simulink model "MicrochipTargetMotorControl"  (R2024b)
settings: Solver=FixedStepDiscrete  StartTime=0.0  StopTime=50  RelTol=1e-3  EnableMultiTasking=on
InitFcn:
  | MicrochipTargetMotorControlData;
  | mcbMotorSwapData;
values from neighbouring files (symbols this model uses):
  Ts = T_pwm    [mcbMotorSwapData.m]
  Ts_motor = T_pwm/2    [mcbMotorSwapData.m]
  Ts_serialIn = 50e-3    (= 0.05)    [MicrochipTargetMotorControlData.m]
  Ts_speed = 10*Ts    [mcbMotorSwapData.m]
undefined symbols (not defined in the file or in its folder): A4, B0, C10, C11, C6, C7, C8, inverter, MaxPer, P17, P20, P39, P40, P41, P43, P44, Pin, pmsm, Resol, s, target, Timer, us
libraries: MCHP_Blockset x19, simulink x13, autolibpmsminterior x1, mcbplantlib x1, mcbcontrolslib x1
(part 1 of 4)
settings Model: ExtModeEnableFloating=off  ExtModeTrigDuration=20  Creator=Lubin Kerhuel  LastModifiedBy=snarayan
settings SolverCC: AlgebraicLoopSolver=TrustRegion
settings OptimizationCC: DefaultParameterBehavior=Inlined  DefaultUnderspecifiedDataType=single  InlineInvariantSignals=on  StrengthReduction=on  PassReuseOutputArgsAs=Individual arguments  ZeroExternalMemoryAtStartup=off  ZeroInternalMemoryAtStartup=off  OptimizeBlockOrder=speed  OptimizationPriority=Speed  OptimizationCustomize=off  MultiThreadedLoops=on  AutoScheduleForLoops=on  EfficientTunableParamExpr=on
settings DebuggingCC: MultiTaskDSMMsg=none  MultiTaskCondExecSysMsg=none  MultiTaskRateTransMsg=warning  ParameterPrecisionLossMsg=none  ParameterTunabilityLossMsg=error  UnconnectedInputMsg=warning  UnconnectedOutputMsg=warning  UnconnectedLineMsg=warning  ArithmeticOperatorsInVariantConditions=warning
settings HardwareCC: ProdBitPerPointer=32  ProdBitPerSizeT=32  ProdBitPerPtrDiffT=32  ProdLargestAtomicInteger=Long  ProdWordSize=32  ProdHWDeviceType=Generic->Custom
settings ModelReferenceCC: ModelReferenceNumInstancesAllowed=Single
settings SFSimCC: MATLABDynamicMemAlloc=off  CustomCodeUndefinedFunction=UseInterfaceOnly
settings RTWCC: Description=Microchip Embedded Target dsPIC33A (real-time)  SystemTargetFile=MCHP_dsPIC33A_stf.tlc  TLCOptions="-aExtModeXCPClassicInterface=0  -aCreateExtModeTypes=1 -aExtModeXCPSimulationTimeInTicks=1"  TemplateMakefile=MCHP_dsPIC33A.tmf  GPUComputeCapability=3.5
settings RTWCC: CustomSourceCode=|
  | void DisablePWMOutputs(void)
  | {
  |     PG3IOCONbits.OVRDAT = 0;
  |     PG2IOCONbits.OVRDAT = 0;
  |     PG1IOCONbits.OVRDAT = 0;
  |     PG3IOCONbits.OVRENH = 1;
  |     PG3IOCONbits.OVRENL = 1;
  |     PG2IOCONbits.OVRENH = 1;
  |     PG2IOCONbits.OVRENL = 1;
  |     PG1IOCONbits.OVRENH = 1;
  |     PG1IOCONbits.OVRENL = 1;
  | }
  | 
  | 
  | void EnablePWMOutputs(void)
  | {
  |     PG3IOCONbits.OVRENH = 0;
  |     PG3IOCONbits.OVRENL = 0;
  |     PG2IOCONbits.OVRENH = 0;
  |     PG2IOCONbits.OVRENL = 0;
  |     PG1IOCONbits.OVRENH = 0;
  |     PG1IOCONbits.OVRENL = 0;
  | }
settings CodeAppCC: ForceParamTrailComments=on  IgnoreCustomStorageClasses=off  MaxIdLength=255  OperatorAnnotations=on  SimulinkDataObjDesc=on  SFDataObjDesc=on  InsertBlockDesc=on
settings STFCustomTargetCC: TargetLibSuffix=_lib.a  TargetLangStandard=C99 (ISO)  MultiwordLength=256  CombineOutputUpdateFcns=on  CombineSignalStateStructs=on  SuppressErrorStatus=on  ERTCustomFileBanners=on  SupportContinuousTime=off  RemoveResetFunc=on  MATLABClassNameForMDSCustomization=Simulink.SoftwareTarget.ERTCustomization  SystemTargetFile=MCHP_dsPIC33A_stf.tlc
settings ERTTargetCC: TargetLibSuffix=_lib.a  TargetLangStandard=C99 (ISO)  ParMdlRefBuildCompliant=off  CompOptLevelCompliant=off  ConcurrentExecutionCompliant=off  CombineSignalStateStructs=on  SuppressErrorStatus=on  SupportNonInlinedSFcns=on  ModelStepFunctionPrototypeControlCompliant=off  CPPClassGenCompliant=off  UseToolchainInfoCompliant=off  ExtModeTransport=1  ExtModeStaticAlloc=on  ExtModeStaticAllocSize=1024  ExtModeMexFile=ext_xcp  ExtModeMexArgs=1 0 460800 './mclv_48v_300w_dspic33ak128mc106_opticalencoder.X/mclv_48v_300w_dspic33ak128mc106_opticalencoder.elf'  ExtModeIntrfLevel=Level2 - Open  ERTSrcFileBannerTemplate=MCHP_dsPIC_code_template.cgt  ERTHdrFileBannerTemplate=MCHP_dsPIC_code_template.cgt  ERTDataSrcFileTemplate=MCHP_dsPIC_code_template.cgt  ERTDataHdrFileTemplate=MCHP_dsPIC_code_template.cgt  ERTCustomFileTemplate=MCHP_main.tlc  MaxLineWidth=110  DynamicArrayContainerType=coder::array

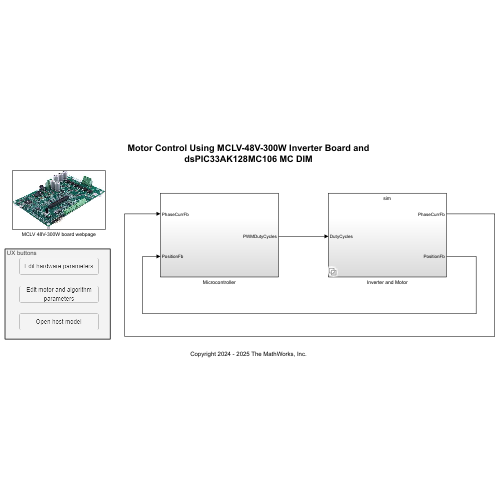
[thumbnail: Simulink's stored preview of the top-level diagram]
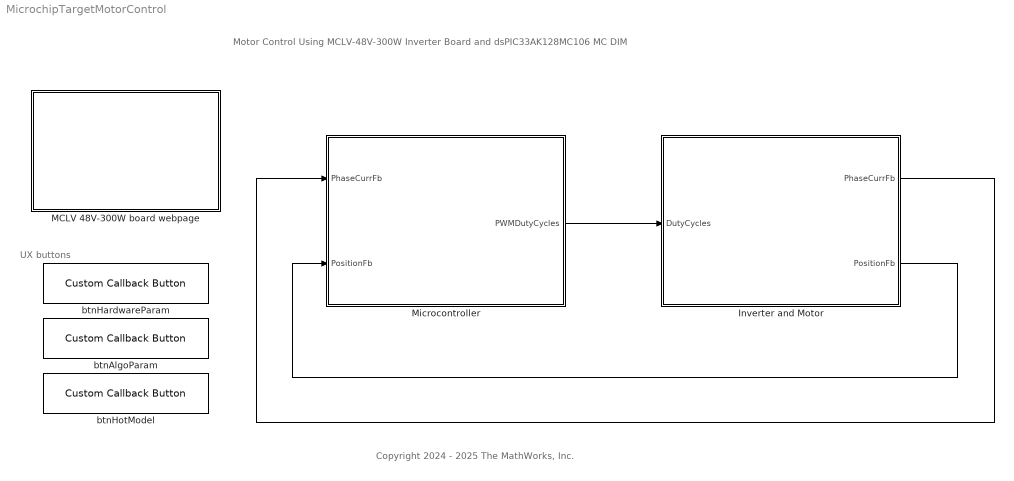
== system MicrochipTargetMotorControl ==
  note: Motor Control Using MCLV-48V-300W Inverter Board and dsPIC33AK128MC106 MC DIM
  note: UX buttons
  note: Copyright 2024 - 2025 The MathWorks, Inc.
  Inverter and Motor : Subsystem  Variant=on  VariantControlMode=sim codegen switching
  MCLV 48V-300W board webpage : Subsystem
      settings: OpenFcn=|
      | web('https://www.microchip.com/en-us/development-tool/EV62P66A','-browser'); % dsPIC33CK256MP508 DIM
      | pause(1);
      | web('https://www.microchip.com/en-us/development-tool/EV18H47A','-browser'); % LVMC 300W
      mask Display: image('MCHP_i_Board_MCLV_300W48V_reduced.jpg');
  Microcontroller : Subsystem
  btnAlgoParam : CustomCallbackButton  Configuration="{\"components\":[{\"name\":\"BackgroundImageComponent\",\"settings\":{\"image\":{\"size\":[0,0],\"src\":\"default\",\"srcOrientation\":\"Right\"},\"position\":[0,0,1,1]}},{\"name\":\"ButtonStateComponent\",\"settings\":{\"buttonType\":\"momentary\",\"clickFcn\":\"edit mcbMotorSwapData.m;\",\"onValue\":1,\"position\":[0,0,1,1],\"pressDelay\":\"500\",\"pressFcn\":\"\",\"repeatInterval\":\"0\",\"states\":[{\"horizontalAlignment\":\"center\",\"image\":{\"position\":[0,0,1,1],\"size\":[1,1],\"src\":\"default\",\"srcOrientation\":\"Right\"},\"label\":{\"color\":[0.01176470588,0.01176470588,0.01176470588,1],\"icon\":{\"size\":[0,0],\"src\":\"default\",\"srcOrientation\":\"Right\"},\"iconPlacement\":\"left\",\"opacity\":1,\"show\":true,\"text\":{\"content\":\"Edit motor and algorithm parameters\",\"font\":\"Helvetica\"}},\"labelOffset\":[0,0],\"verticalAlignment\":\"middle\"},{\"horizontalAlignment\":\"center\",\"image\":{\"position\":[0,0,1,1],\"size\":[1,1],\"src\":\"default\",\"srcOrientation\":\"Right\"},\"label\":{\"color\":[0.01176470588,0.01176470588,0.01176470588,1],\"icon\":{\"size\":[0,0],\"src\":\"default\",\"srcOrientation\":\"Right\"},\"iconPlacement\":\"left\",\"opacity\":1,\"show\":true,\"text\":{\"content\":\"Edit motor and algorithm parameters\",\"font\":\"Helvetica\"}},\"labelOffset\":[0,0],\"verticalAlignment\":\"middle\"},{\"horizontalAlignment\":\"center\",\"image\":{\"position\":[0,0,1,1],\"size\":[1,1],\"src\":\"default\",\"srcOrientation\":\"Right\"},\"label\":{\"color\":[0.01176470588,0.01176470588,0.01176470588,1],\"icon\":{\"size\":[0,0],\"src\":\"default\",\"srcOrientation\":\"Right\"},\"iconPlacement\":\"left\",\"opacity\":1,\"show\":true,\"text\":{\"content\":\"Edit motor and algorithm parameters\",\"font\":\"Helvetica\"}},\"labelOffset\":[0,0],\"verticalAlignment\":\"middle\"},{\"horizontalAlignment\":\"center\",\"image\":{\"position\":[0,0,1,1],\"size\":[1,1],\"src\":\"default\",\"srcOrientation\":\"Right\"},\"label\":{\"color\":[0.01176470588,0.01176470588,0.01176470588,1],\"icon\":{\"size\":[0,0],\"src\":\"default\",\"srcOrientation\":\"Right\"},\"iconPlacement\":\"left\",\"opacity\":1,\"show\":true,\"text\":{\"content\":\"Edit motor and algorithm parameters\",\"font\":\"Helvetica\"}},\"labelOffset\":[0,0],\"verticalAlignment\":\"middle\"}]}},{\"name\":\"ForegroundImageComponent\",\"settings\":{\"image\":{\"size\":[0,0],\"src\":\"default\",\"srcOrientation\":\"Right\"},\"isForeground\":1,\"position\":[0,0,1,1]}}],\"settings\":{\"BindingType\":\"standalone\",\"backgroundColor\":[244,244,244,1],\"backgroundOffset\":0.2,\"backgroundOpacity\":1,\"fixedAspectRatio\":\"off\",\"foregroundColor\":[0.01176470588,0.01176470588,0.01176470588,1],\"migratedFromLegacy\":true,\"useBackgroundColor\":true,\"variant\":\"callback\",\"version\":\"R2024b\"},\"type\":\"Button\"}"  CustomBackgroundColor="{\"color\":[0.9568627451,0.9568627451,0.9568627451],\"show\":true}"
  btnHardwareParam : CustomCallbackButton  Configuration="{\"components\":[{\"name\":\"BackgroundImageComponent\",\"settings\":{\"image\":{\"size\":[0,0],\"src\":\"default\",\"srcOrientation\":\"Right\"},\"position\":[0,0,1,1]}},{\"name\":\"ButtonStateComponent\",\"settings\":{\"buttonType\":\"momentary\",\"clickFcn\":\"edit MicrochipTargetMotorControlData.m;\",\"onValue\":1,\"position\":[0,0,1,1],\"pressDelay\":\"500\",\"pressFcn\":\"\",\"repeatInterval\":\"0\",\"states\":[{\"horizontalAlignment\":\"center\",\"image\":{\"position\":[0,0,1,1],\"size\":[1,1],\"src\":\"default\",\"srcOrientation\":\"Right\"},\"label\":{\"color\":[0.01176470588,0.01176470588,0.01176470588,1],\"icon\":{\"size\":[0,0],\"src\":\"default\",\"srcOrientation\":\"Right\"},\"iconPlacement\":\"left\",\"opacity\":1,\"show\":true,\"text\":{\"content\":\"Edit hardware parameters\",\"font\":\"Helvetica\"}},\"labelOffset\":[0,0],\"verticalAlignment\":\"middle\"},{\"horizontalAlignment\":\"center\",\"image\":{\"position\":[0,0,1,1],\"size\":[1,1],\"src\":\"default\",\"srcOrientation\":\"Right\"},\"label\":{\"color\":[0.01176470588,0.01176470588,0.01176470588,1],\"icon\":{\"size\":[0,0],\"src\":\"default\",\"srcOrientation\":\"Right\"},\"iconPlacement\":\"left\",\"opacity\":1,\"show\":true,\"text\":{\"content\":\"Edit hardware parameters\",\"font\":\"Helvetica\"}},\"labelOffset\":[0,0],\"verticalAlignment\":\"middle\"},{\"horizontalAlignment\":\"center\",\"image\":{\"position\":[0,0,1,1],\"size\":[1,1],\"src\":\"default\",\"srcOrientation\":\"Right\"},\"label\":{\"color\":[0.01176470588,0.01176470588,0.01176470588,1],\"icon\":{\"size\":[0,0],\"src\":\"default\",\"srcOrientation\":\"Right\"},\"iconPlacement\":\"left\",\"opacity\":1,\"show\":true,\"text\":{\"content\":\"Edit hardware parameters\",\"font\":\"Helvetica\"}},\"labelOffset\":[0,0],\"verticalAlignment\":\"middle\"},{\"horizontalAlignment\":\"center\",\"image\":{\"position\":[0,0,1,1],\"size\":[1,1],\"src\":\"default\",\"srcOrientation\":\"Right\"},\"label\":{\"color\":[0.01176470588,0.01176470588,0.01176470588,1],\"icon\":{\"size\":[0,0],\"src\":\"default\",\"srcOrientation\":\"Right\"},\"iconPlacement\":\"left\",\"opacity\":1,\"show\":true,\"text\":{\"content\":\"Edit hardware parameters\",\"font\":\"Helvetica\"}},\"labelOffset\":[0,0],\"verticalAlignment\":\"middle\"}]}},{\"name\":\"ForegroundImageComponent\",\"settings\":{\"image\":{\"size\":[0,0],\"src\":\"default\",\"srcOrientation\":\"Right\"},\"isForeground\":1,\"position\":[0,0,1,1]}}],\"settings\":{\"BindingType\":\"standalone\",\"backgroundColor\":[244,244,244,1],\"backgroundOffset\":0.2,\"backgroundOpacity\":1,\"fixedAspectRatio\":\"off\",\"foregroundColor\":[0.01176470588,0.01176470588,0.01176470588,1],\"migratedFromLegacy\":true,\"useBackgroundColor\":true,\"variant\":\"callback\",\"version\":\"R2024b\"},\"type\":\"Button\"}"  CustomBackgroundColor="{\"color\":[0.9568627451,0.9568627451,0.9568627451],\"show\":true}"
  btnHotModel : CustomCallbackButton  Configuration="{\"components\":[{\"name\":\"BackgroundImageComponent\",\"settings\":{\"image\":{\"size\":[0,0],\"src\":\"default\",\"srcOrientation\":\"Right\"},\"position\":[0,0,1,1]}},{\"name\":\"ButtonStateComponent\",\"settings\":{\"buttonType\":\"momentary\",\"clickFcn\":\"MicrochipHostMotorControl;\",\"onValue\":1,\"position\":[0,0,1,1],\"pressDelay\":\"500\",\"pressFcn\":\"\",\"repeatInterval\":\"0\",\"states\":[{\"horizontalAlignment\":\"center\",\"image\":{\"position\":[0,0,1,1],\"size\":[1,1],\"src\":\"default\",\"srcOrientation\":\"Right\"},\"label\":{\"color\":[0.01176470588,0.01176470588,0.01176470588,1],\"icon\":{\"size\":[0,0],\"src\":\"default\",\"srcOrientation\":\"Right\"},\"iconPlacement\":\"left\",\"opacity\":1,\"show\":true,\"text\":{\"content\":\"Open host model\",\"font\":\"Helvetica\"}},\"labelOffset\":[0,0],\"verticalAlignment\":\"middle\"},{\"horizontalAlignment\":\"center\",\"image\":{\"position\":[0,0,1,1],\"size\":[1,1],\"src\":\"default\",\"srcOrientation\":\"Right\"},\"label\":{\"color\":[0.01176470588,0.01176470588,0.01176470588,1],\"icon\":{\"size\":[0,0],\"src\":\"default\",\"srcOrientation\":\"Right\"},\"iconPlacement\":\"left\",\"opacity\":1,\"show\":true,\"text\":{\"content\":\"Open host model\",\"font\":\"Helvetica\"}},\"labelOffset\":[0,0],\"verticalAlignment\":\"middle\"},{\"horizontalAlignment\":\"center\",\"image\":{\"position\":[0,0,1,1],\"size\":[1,1],\"src\":\"default\",\"srcOrientation\":\"Right\"},\"label\":{\"color\":[0.01176470588,0.01176470588,0.01176470588,1],\"icon\":{\"size\":[0,0],\"src\":\"default\",\"srcOrientation\":\"Right\"},\"iconPlacement\":\"left\",\"opacity\":1,\"show\":true,\"text\":{\"content\":\"Open host model\",\"font\":\"Helvetica\"}},\"labelOffset\":[0,0],\"verticalAlignment\":\"middle\"},{\"horizontalAlignment\":\"center\",\"image\":{\"position\":[0,0,1,1],\"size\":[1,1],\"src\":\"default\",\"srcOrientation\":\"Right\"},\"label\":{\"color\":[0.01176470588,0.01176470588,0.01176470588,1],\"icon\":{\"size\":[0,0],\"src\":\"default\",\"srcOrientation\":\"Right\"},\"iconPlacement\":\"left\",\"opacity\":1,\"show\":true,\"text\":{\"content\":\"Open host model\",\"font\":\"Helvetica\"}},\"labelOffset\":[0,0],\"verticalAlignment\":\"middle\"}]}},{\"name\":\"ForegroundImageComponent\",\"settings\":{\"image\":{\"size\":[0,0],\"src\":\"default\",\"srcOrientation\":\"Right\"},\"isForeground\":1,\"position\":[0,0,1,1]}}],\"settings\":{\"BindingType\":\"standalone\",\"backgroundColor\":[244,244,244,1],\"backgroundOffset\":0.2,\"backgroundOpacity\":1,\"fixedAspectRatio\":\"off\",\"foregroundColor\":[0.01176470588,0.01176470588,0.01176470588,1],\"migratedFromLegacy\":true,\"useBackgroundColor\":true,\"variant\":\"callback\",\"version\":\"R2024b\"},\"type\":\"Button\"}"  CustomBackgroundColor="{\"color\":[0.9568627451,0.9568627451,0.9568627451],\"show\":true}"
  wires:
  Microcontroller/1(PWMDutyCycles) -> Inverter and Motor/1(DutyCycles)
  Inverter and Motor/1(PhaseCurrFb) -> Microcontroller/1(PhaseCurrFb)
  Inverter and Motor/2(PositionFb) -> Microcontroller/2(PositionFb)

== system MicrochipTargetMotorControl/Inverter and Motor ==
  DutyCycles : Inport
  codegen : Subsystem  VariantControl=(codegen)
  sim : Subsystem  VariantControl=(sim)
  PhaseCurrFb : Outport
  PositionFb : Outport  Port=2

== system MicrochipTargetMotorControl/MCLV 48V-300W board webpage ==

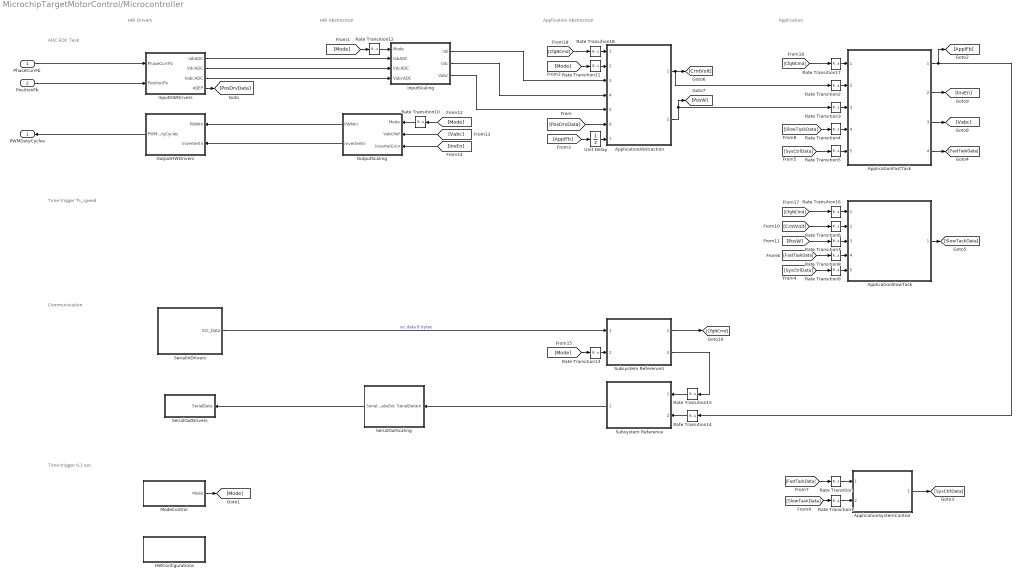
== system MicrochipTargetMotorControl/Microcontroller ==
  note: ADC EOC Task
  note: HW Drivers
  note: HW Abstraction
  note: Application Abstraction
  note: Application
  note: Time trigger Ts_speed
  note: Communication
  note: Time trigger 0.1 sec
  PhaseCurrFb : Inport
  PositionFb : Inport  Port=2
  ApplicationAbstraction : Subsystem  ReferencedSubsystem=ApplicationAbstractionMotorSwap
  ApplicationFastTask : Subsystem  TreatAsAtomicUnit=on  SystemSampleTime=Ts  ReferencedSubsystem=ApplicationMotorSwapHighPrio
  ApplicationSlowTask : Subsystem  TreatAsAtomicUnit=on  SystemSampleTime=Ts_speed  ReferencedSubsystem=ApplicationMotorSwapLowPrio
  ApplicationSystemControl : Subsystem  TreatAsAtomicUnit=on  SystemSampleTime=0.1  ReferencedSubsystem=ApplicationMotorSwapSysControl
  HWConfigurations : Subsystem
  InputHWDrivers : Subsystem  Variant=on  VariantControlMode=sim codegen switching
  InputScaling : Subsystem
  ModeControl : Subsystem  Variant=on
  OutputHWDrivers : Subsystem  Variant=on  VariantControlMode=sim codegen switching
  OutputScaling : Subsystem
  Rate Transition{,1..10,12,16..17} (14 alike) : RateTransition  Deterministic=off
  Rate Transition11 : RateTransition  Deterministic=off  OutPortSampleTime=Ts
  Rate Transition13 : RateTransition  Deterministic=off  OutPortSampleTime=Ts_serialIn
  Rate Transition14 : RateTransition  Deterministic=off  OutPortSampleTime=Ts_serialOut
  Rate Transition15 : RateTransition  Deterministic=off  OutPortSampleTime=Ts_serialOut
  Rate Transition18 : RateTransition  Deterministic=off  OutPortSampleTime=Ts
  SerialInDrivers : Subsystem
  SerialOutDrivers : Subsystem  Variant=on  VariantControlMode=sim codegen switching
  SerialOutScaling : Subsystem
  Subsystem Reference : Subsystem  TreatAsAtomicUnit=on  ReferencedSubsystem=SCIOutAbstractionMotorSwap
  Subsystem Reference1 : Subsystem  TreatAsAtomicUnit=on  ReferencedSubsystem=SCIInAbstractionMotorSwap
  Unit Delay : UnitDelay  SampleTime=-1  HasFrameUpgradeWarning=on
  PWMDutyCycles : Outport
  wires:
  PositionFb/1 -> InputHWDrivers/2(PositionFb)
  PhaseCurrFb/1 -> InputHWDrivers/1(PhaseCurrFb)
  OutputHWDrivers/1(PWMDutyCycles) -> PWMDutyCycles/1
  InputHWDrivers/1(IabADC) -> InputScaling/2(IabADC)
  InputHWDrivers/2(VdcADC) -> InputScaling/3(VdcADC)
  InputHWDrivers/3(VabcADC) -> InputScaling/4(VabcADC)
  OutputScaling/1(PWMIn) -> OutputHWDrivers/1(PWMIn)
  OutputScaling/2(InverterEn) -> OutputHWDrivers/2(InverterEn)
  InputScaling/1(Iab) -> ApplicationAbstraction/3
  InputScaling/2(Vdc) -> ApplicationAbstraction/4
  InputScaling/3(Vabc) -> ApplicationAbstraction/5
  InputHWDrivers/4(eQEP) -> [PosDrvData]
  [PosDrvData] -> ApplicationAbstraction/6
  ModeControl/1(Mode) -> [Mode]
  [Mode] -> Rate Transition12/1
  [Mode] -> Rate Transition11/1
  ApplicationFastTask/1 -> [ApplFb], Rate Transition14/1
  [ApplFb] -> Unit Delay/1
  Unit Delay/1 -> ApplicationAbstraction/7
  ApplicationSystemControl/1 -> [SysCtrlData]
  [SysCtrlData] -> Rate Transition9/1
  [SysCtrlData] -> Rate Transition5/1
  ApplicationFastTask/4 -> [FastTaskData]
  [FastTaskData] -> Rate Transition8/1
  [FastTaskData] -> Rate Transition/1
  ApplicationSlowTask/1 -> [SlowTaskData]
  [SlowTaskData] -> Rate Transition1/1
  ApplicationAbstraction/1 -> Rate Transition2/1, [CrntVolt]
  [CrntVolt] -> Rate Transition6/1
  ApplicationAbstraction/2 -> [PosW], Rate Transition3/1
  [PosW] -> Rate Transition7/1
  [Mode] -> Rate Transition10/1
  ApplicationFastTask/3 -> [Vabc]
  [Vabc] -> OutputScaling/2(VabcRef)
  ApplicationFastTask/2 -> [InvEn]
  [InvEn] -> OutputScaling/3(InverterEnIn)
  Rate Transition/1 -> ApplicationSystemControl/1
  Rate Transition1/1 -> ApplicationSystemControl/2
  Rate Transition2/1 -> ApplicationFastTask/2
  Rate Transition3/1 -> ApplicationFastTask/3
  [SlowTaskData] -> Rate Transition4/1
  Rate Transition4/1 -> ApplicationFastTask/4
  Rate Transition5/1 -> ApplicationFastTask/5
  Rate Transition10/1 -> OutputScaling/1(Mode)
  Rate Transition11/1 -> ApplicationAbstraction/2
  Rate Transition12/1 -> InputScaling/1(Mode)
  Subsystem Reference/1 -> SerialOutScaling/1(SerialDataIn)
  SerialOutScaling/1(SerialDataOut) -> SerialOutDrivers/1(SerialData)
  [Mode] -> Rate Transition13/1
  Rate Transition13/1 -> Subsystem Reference1/2
  SerialInDrivers/1(SCI_Data) -> Subsystem Reference1/1  "sci data 8 bytes"
  Rate Transition14/1 -> Subsystem Reference/2
  Rate Transition15/1 -> Subsystem Reference/1
  Subsystem Reference1/2 -> Rate Transition15/1
  Rate Transition6/1 -> ApplicationSlowTask/2
  Rate Transition7/1 -> ApplicationSlowTask/3
  Rate Transition8/1 -> ApplicationSlowTask/4
  Rate Transition9/1 -> ApplicationSlowTask/5
  Subsystem Reference1/1 -> [CfgNCmd]
  Rate Transition16/1 -> ApplicationSlowTask/1
  [CfgNCmd] -> Rate Transition16/1
  [CfgNCmd] -> Rate Transition17/1
  Rate Transition17/1 -> ApplicationFastTask/1
  [CfgNCmd] -> Rate Transition18/1
  Rate Transition18/1 -> ApplicationAbstraction/1

== system MicrochipTargetMotorControl/Inverter and Motor/codegen ==
  DutyCycles : Inport
  Ground : Ground
  Terminator : Terminator
  PhaseCurrFb : Outport
  PositionFb : Outport  Port=2
  wires:
  DutyCycles/1 -> Terminator/1
  Ground/1 -> PhaseCurrFb/1, PositionFb/1

== system MicrochipTargetMotorControl/Inverter and Motor/sim ==
  DutyCycles : Inport
  Motor : Subsystem
  Sensor_Measurements : Subsystem
  PhaseCurrFb : Outport
  PositionFb : Outport  Port=2
  wires:
  Motor/2(ThetaMech) -> Sensor_Measurements/2(ThetaMech)
  Motor/1(Iabc) -> Sensor_Measurements/1(Iabc)
  DutyCycles/1 -> Motor/1(Duty_Cycles)
  Sensor_Measurements/1(Iab_fb) -> PhaseCurrFb/1
  Sensor_Measurements/2(Pos_fb) -> PositionFb/1
